simulink model "PHIL_DHS_DQ_Control"  (R2019b)
settings: Solver=VariableStepAuto  StartTime=0.0  StopTime=00.5  RelTol=1e-3
undefined symbols (not defined in the file): Apd_i_dhs, Apd_u_dhs, C_dhs, f_sw_dhs, L_dhs, Tid_i_dhs, Tid_u_dhs, U_DC
libraries: coordinate_transformations x8, simulink x4
settings Model: Creator=kissd  LastModifiedBy=kissd

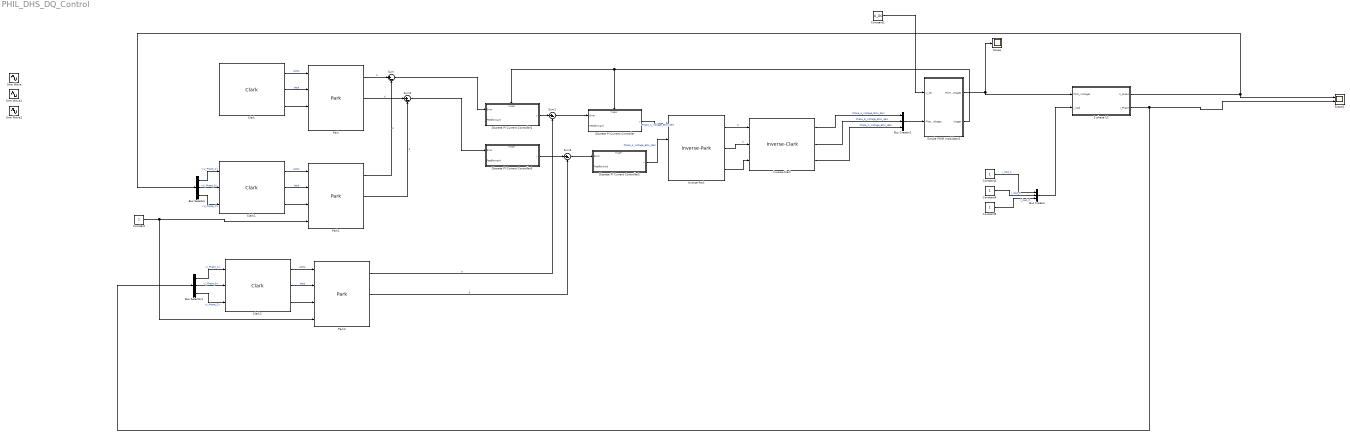
== system PHIL_DHS_DQ_Control ==
  3 phase LC : Subsystem
  Bus Creator : BusCreator  Inputs=3
  Bus Creator1 : BusCreator  Inputs=3
  Bus Selector : BusSelector  OutputSignals=U_Phase_A,U_Phase_B,U_Phase_C
  Bus Selector1 : BusSelector  OutputSignals=I_Phase_A,I_Phase_B,I_Phase_C
  Clark : coordinate_transformations/Clark  SystemSampleTime=-1  Latency=0  AutoFrameSizeCalculation=off
  Clark1 : coordinate_transformations/Clark  SystemSampleTime=-1  Latency=0  AutoFrameSizeCalculation=off
  Clark2 : coordinate_transformations/Clark  SystemSampleTime=-1  Latency=0  AutoFrameSizeCalculation=off
  Constant{,3..5} (4 alike) : Constant
  Constant1 : Constant  Value=U_DC
  Discrete PI Current Controller : Subsystem  AncestorBlock=controllers/Discrete PI Controller  mask(Continous PI Controller){Apd=Apd_i_dhs, Tid=Tid_i_dhs, fs=f_sw_dhs, UpperSat=U_DC, LowerSat=0}
      mask prompts: Apd "Proprotional Gain"; Tid "Integration Time"; fs "fsw"; UpperSat "Max. Saturation"; LowerSat "Min. Saturation"
      mask help: Continous PI Controller description.
  Discrete PI Current Controller1 : Subsystem  AncestorBlock=controllers/Discrete PI Controller  mask(Continous PI Controller){Apd=Apd_u_dhs, Tid=Tid_u_dhs, fs=f_sw_dhs, UpperSat=200, LowerSat=-200}
      mask prompts: Apd "Proprotional Gain"; Tid "Integration Time"; fs "fsw"; UpperSat "Max. Saturation"; LowerSat "Min. Saturation"
      mask help: Continous PI Controller description.
  Discrete PI Current Controller2 : Subsystem  AncestorBlock=controllers/Discrete PI Controller  mask(Continous PI Controller){Apd=Apd_i_dhs, Tid=Tid_i_dhs, fs=f_sw_dhs, UpperSat=U_DC, LowerSat=0}
      mask prompts: Apd "Proprotional Gain"; Tid "Integration Time"; fs "fsw"; UpperSat "Max. Saturation"; LowerSat "Min. Saturation"
      mask help: Continous PI Controller description.
  Discrete PI Current Controller3 : Subsystem  AncestorBlock=controllers/Discrete PI Controller  mask(Continous PI Controller){Apd=Apd_u_dhs, Tid=Tid_u_dhs, fs=f_sw_dhs, UpperSat=200, LowerSat=-200}
      mask prompts: Apd "Proprotional Gain"; Tid "Integration Time"; fs "fsw"; UpperSat "Max. Saturation"; LowerSat "Min. Saturation"
      mask help: Continous PI Controller description.
  Inverse-Clark : coordinate_transformations/Inverse-Clark  SystemSampleTime=-1  Latency=0  AutoFrameSizeCalculation=off
  Inverse-Park : coordinate_transformations/Inverse-Park  SystemSampleTime=-1  Latency=0  AutoFrameSizeCalculation=off
  Park : coordinate_transformations/Park  SystemSampleTime=-1  Latency=0  AutoFrameSizeCalculation=off
  Park1 : coordinate_transformations/Park  SystemSampleTime=-1  Latency=0  AutoFrameSizeCalculation=off
  Park2 : coordinate_transformations/Park  SystemSampleTime=-1  Latency=0  AutoFrameSizeCalculation=off
  Scope : Scope
  Scope2 : Scope  NumInputPorts=2
  Simple PWM modulator2 : Subsystem  AncestorBlock=controllers/Simple PWM modulator
  Sine Wave : Sin  SampleTime=0
  Sine Wave1 : Sin  SampleTime=0
  Sine Wave2 : Sin  SampleTime=0
  Sum{,1..3} (4 alike) : Sum  Inputs=|+-
  wires:
  Constant1/1 -> Simple PWM modulator2/1(U_DC)
  Inverse-Clark/3 -> Bus Creator1/3  "Phase_C_Voltage_EMU_dem"
  Inverse-Clark/2 -> Bus Creator1/2  "Phase_B_Voltage_EMU_dem"
  Sum1/1 -> Discrete PI Current Controller/1(Error)
  Inverse-Clark/1 -> Bus Creator1/1  "Phase_A_Voltage_EMU_dem"
  Simple PWM modulator2/1(PWM_Voltages) -> Scope/1, 3 phase LC/1(PWM_Voltages)
  Bus Creator1/1 -> Simple PWM modulator2/2(Phase_Voltages)
  Simple PWM modulator2/2(trigger) -> Discrete PI Current Controller1/Trigger, Discrete PI Current Controller/Trigger
  Discrete PI Current Controller1/1(y) -> Sum1/1
  Sum/1 -> Discrete PI Current Controller1/1(Error)
  Clark/1 -> Park/1  "alpha"
  Clark/2 -> Park/2  "beta"
  Clark/3 -> Park/3
  3 phase LC/2(I_Phase) -> Bus Selector1/1, Scope2/2
  3 phase LC/1(U_phase) -> Scope2/1, Bus Selector/1
  Constant3/1 -> Bus Creator/1  "I_load_A"
  Constant4/1 -> Bus Creator/2  "I_load_B"
  Constant5/1 -> Bus Creator/3  "I_load_C"
  Bus Creator/1 -> 3 phase LC/2(I_load)
  Inverse-Park/1 -> Inverse-Clark/1  "d"
  Inverse-Park/2 -> Inverse-Clark/2  "q"
  Inverse-Park/3 -> Inverse-Clark/3
  Park/1 -> Sum/1  "d"
  Discrete PI Current Controller/1(y) -> Inverse-Park/1  "Phase_A_Voltage_EMU_dem"
  Sum2/1 -> Discrete PI Current Controller3/1(Error)
  Discrete PI Current Controller3/1(y) -> Sum3/1
  Park/2 -> Sum2/1  "d"
  Sum3/1 -> Discrete PI Current Controller2/1(Error)
  Discrete PI Current Controller2/1(y) -> Inverse-Park/2  "Phase_A_Voltage_EMU_dem"
  Clark1/3 -> Park1/3
  Clark1/1 -> Park1/1  "alpha"
  Clark1/2 -> Park1/2  "beta"
  Clark2/3 -> Park2/3
  Clark2/1 -> Park2/1  "alpha"
  Clark2/2 -> Park2/2  "beta"
  Bus Selector/1 -> Clark1/1  "<U_Phase_A>"
  Bus Selector/2 -> Clark1/2  "<U_Phase_B>"
  Bus Selector/3 -> Clark1/3  "<U_Phase_C>"
  Bus Selector1/1 -> Clark2/1  "<I_Phase_A>"
  Bus Selector1/2 -> Clark2/2  "<I_Phase_B>"
  Bus Selector1/3 -> Clark2/3  "<I_Phase_C>"
  Constant/1 -> Park2/4, Park1/4
  Park1/1 -> Sum/2  "d"
  Park1/2 -> Sum2/2  "d"
  Park2/1 -> Sum1/2  "d"
  Park2/2 -> Sum3/2  "d"

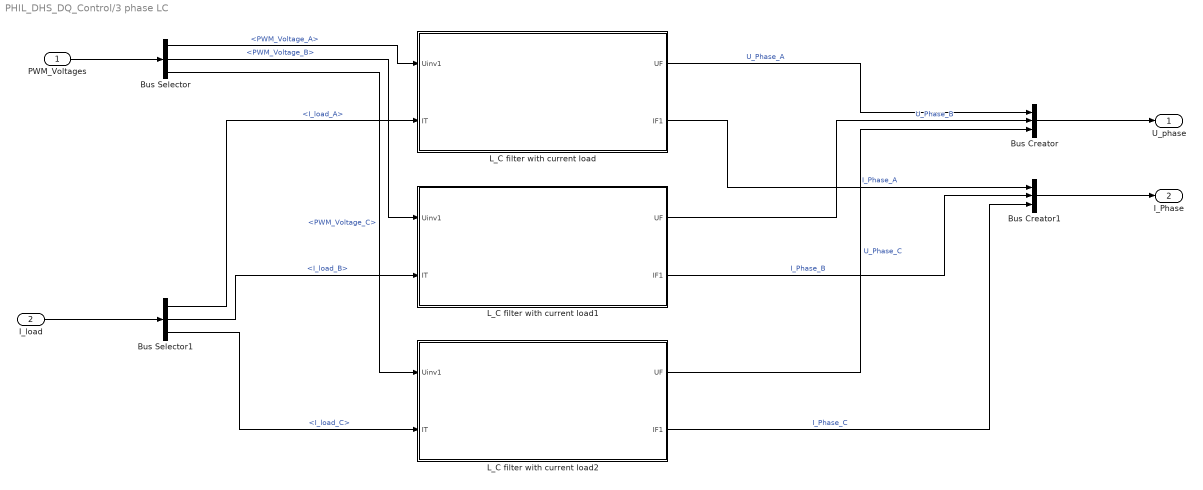
== system PHIL_DHS_DQ_Control/3 phase LC ==
  PWM_Voltages : Inport
  I_load : Inport  Port=2
  Bus Creator : BusCreator  Inputs=3
  Bus Creator1 : BusCreator  Inputs=3
  Bus Selector : BusSelector  OutputSignals=PWM_Voltage_A,PWM_Voltage_B,PWM_Voltage_C
  Bus Selector1 : BusSelector  OutputSignals=I_load_A,I_load_B,I_load_C
  L_C filter with current load : Subsystem
  L_C filter with current load1 : Subsystem
  L_C filter with current load2 : Subsystem
  U_phase : Outport
  I_Phase : Outport  Port=2
  wires:
  L_C filter with current load1/1(UF) -> Bus Creator/2  "U_Phase_B"
  L_C filter with current load2/1(UF) -> Bus Creator/3  "U_Phase_C"
  Bus Selector1/3 -> L_C filter with current load2/2(IT)  "<I_load_C>"
  L_C filter with current load1/2(IF1) -> Bus Creator1/2  "I_Phase_B"
  L_C filter with current load2/2(IF1) -> Bus Creator1/3  "I_Phase_C"
  PWM_Voltages/1 -> Bus Selector/1
  Bus Selector/1 -> L_C filter with current load/1(Uinv1)  "<PWM_Voltage_A>"
  Bus Selector/2 -> L_C filter with current load1/1(Uinv1)  "<PWM_Voltage_B>"
  Bus Selector/3 -> L_C filter with current load2/1(Uinv1)  "<PWM_Voltage_C>"
  Bus Creator/1 -> U_phase/1
  L_C filter with current load/1(UF) -> Bus Creator/1  "U_Phase_A"
  L_C filter with current load/2(IF1) -> Bus Creator1/1  "I_Phase_A"
  Bus Creator1/1 -> I_Phase/1
  I_load/1 -> Bus Selector1/1
  Bus Selector1/1 -> L_C filter with current load/2(IT)  "<I_load_A>"
  Bus Selector1/2 -> L_C filter with current load1/2(IT)  "<I_load_B>"

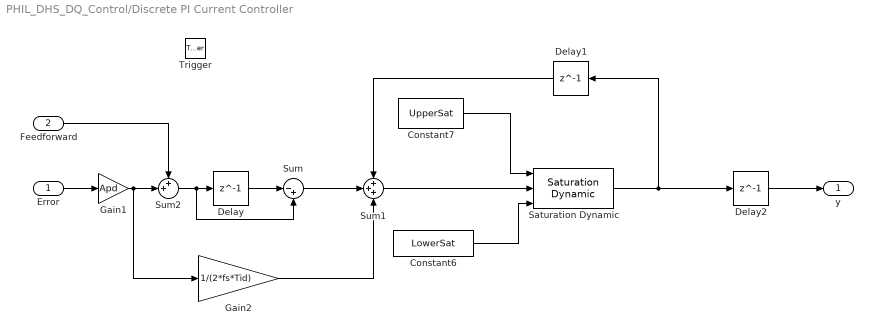
== system PHIL_DHS_DQ_Control/Discrete PI Current Controller ==
  Error : Inport
  Feedforward : Inport  Port=2
  Trigger : TriggerPort  TriggerType=either  VariantControl=Variant  PortDimensions=1
  Constant6 : Constant  Value=LowerSat
  Constant7 : Constant  Value=UpperSat
  Delay : Delay  DelayLength=1
  Delay1 : Delay  DelayLength=1
  Delay2 : Delay  DelayLength=1
  Gain1 : Gain  Gain=Apd
  Gain2 : Gain  Gain=1/(2*fs*Tid)
  Saturation Dynamic : simulink/Discontinuities/Saturation Dynamic  OutMin=[]  OutMax=[]  OutDataTypeStr=Inherit: Same as second input  OutDataType=fixdt(1, 16)  OutScaling=2^-10  DoSatur=off
  Sum : Sum  Inputs=|-+
  Sum1 : Sum  Inputs=+++
  Sum2 : Sum  Inputs=++|
  y : Outport
  wires:
  Error/1 -> Gain1/1
  Gain1/1 -> Sum2/2, Gain2/1
  Sum1/1 -> Saturation Dynamic/2
  Saturation Dynamic/1 -> Delay1/1, Delay2/1
  Constant7/1 -> Saturation Dynamic/1
  Constant6/1 -> Saturation Dynamic/3
  Delay/1 -> Sum/1
  Sum/1 -> Sum1/2
  Gain2/1 -> Sum1/3
  Delay1/1 -> Sum1/1
  Delay2/1 -> y/1
  Sum2/1 -> Sum/2, Delay/1
  Feedforward/1 -> Sum2/1

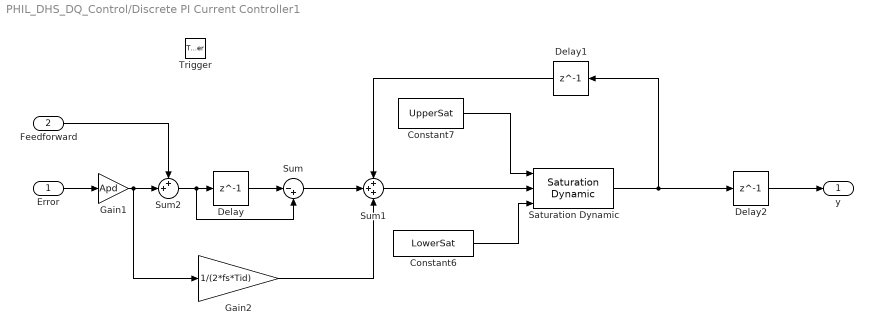
== system PHIL_DHS_DQ_Control/Discrete PI Current Controller1 ==
  Error : Inport
  Feedforward : Inport  Port=2
  Trigger : TriggerPort  TriggerType=either  VariantControl=Variant  PortDimensions=1
  Constant6 : Constant  Value=LowerSat
  Constant7 : Constant  Value=UpperSat
  Delay : Delay  DelayLength=1
  Delay1 : Delay  DelayLength=1
  Delay2 : Delay  DelayLength=1
  Gain1 : Gain  Gain=Apd
  Gain2 : Gain  Gain=1/(2*fs*Tid)
  Saturation Dynamic : simulink/Discontinuities/Saturation Dynamic  OutMin=[]  OutMax=[]  OutDataTypeStr=Inherit: Same as second input  OutDataType=fixdt(1, 16)  OutScaling=2^-10  DoSatur=off
  Sum : Sum  Inputs=|-+
  Sum1 : Sum  Inputs=+++
  Sum2 : Sum  Inputs=++|
  y : Outport
  wires:
  Error/1 -> Gain1/1
  Gain1/1 -> Sum2/2, Gain2/1
  Sum1/1 -> Saturation Dynamic/2
  Saturation Dynamic/1 -> Delay1/1, Delay2/1
  Constant7/1 -> Saturation Dynamic/1
  Constant6/1 -> Saturation Dynamic/3
  Delay/1 -> Sum/1
  Sum/1 -> Sum1/2
  Gain2/1 -> Sum1/3
  Delay1/1 -> Sum1/1
  Delay2/1 -> y/1
  Sum2/1 -> Sum/2, Delay/1
  Feedforward/1 -> Sum2/1

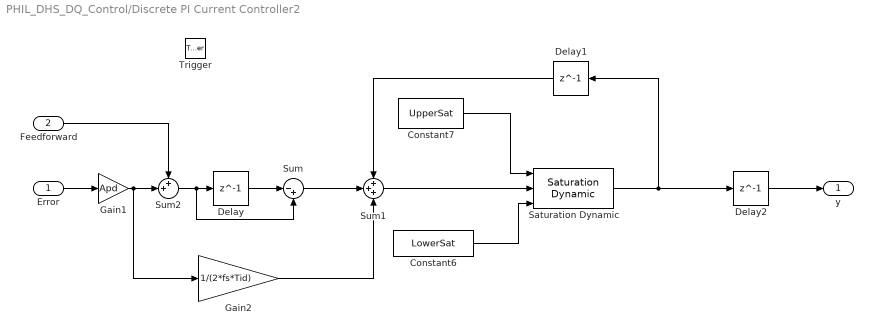
== system PHIL_DHS_DQ_Control/Discrete PI Current Controller2 ==
  Error : Inport
  Feedforward : Inport  Port=2
  Trigger : TriggerPort  TriggerType=either  VariantControl=Variant  PortDimensions=1
  Constant6 : Constant  Value=LowerSat
  Constant7 : Constant  Value=UpperSat
  Delay : Delay  DelayLength=1
  Delay1 : Delay  DelayLength=1
  Delay2 : Delay  DelayLength=1
  Gain1 : Gain  Gain=Apd
  Gain2 : Gain  Gain=1/(2*fs*Tid)
  Saturation Dynamic : simulink/Discontinuities/Saturation Dynamic  OutMin=[]  OutMax=[]  OutDataTypeStr=Inherit: Same as second input  OutDataType=fixdt(1, 16)  OutScaling=2^-10  DoSatur=off
  Sum : Sum  Inputs=|-+
  Sum1 : Sum  Inputs=+++
  Sum2 : Sum  Inputs=++|
  y : Outport
  wires:
  Error/1 -> Gain1/1
  Gain1/1 -> Sum2/2, Gain2/1
  Sum1/1 -> Saturation Dynamic/2
  Saturation Dynamic/1 -> Delay1/1, Delay2/1
  Constant7/1 -> Saturation Dynamic/1
  Constant6/1 -> Saturation Dynamic/3
  Delay/1 -> Sum/1
  Sum/1 -> Sum1/2
  Gain2/1 -> Sum1/3
  Delay1/1 -> Sum1/1
  Delay2/1 -> y/1
  Sum2/1 -> Sum/2, Delay/1
  Feedforward/1 -> Sum2/1

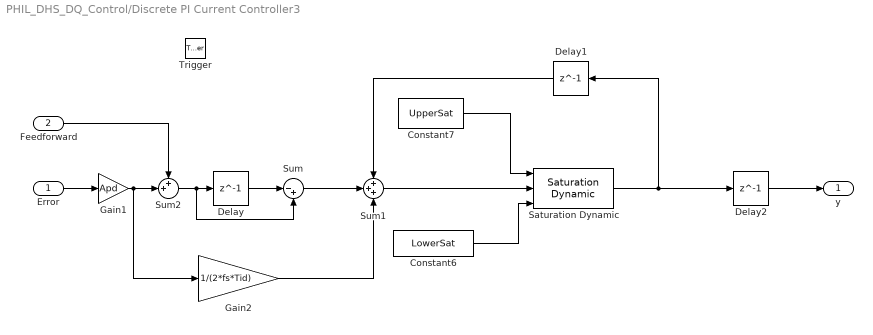
== system PHIL_DHS_DQ_Control/Discrete PI Current Controller3 ==
  Error : Inport
  Feedforward : Inport  Port=2
  Trigger : TriggerPort  TriggerType=either  VariantControl=Variant  PortDimensions=1
  Constant6 : Constant  Value=LowerSat
  Constant7 : Constant  Value=UpperSat
  Delay : Delay  DelayLength=1
  Delay1 : Delay  DelayLength=1
  Delay2 : Delay  DelayLength=1
  Gain1 : Gain  Gain=Apd
  Gain2 : Gain  Gain=1/(2*fs*Tid)
  Saturation Dynamic : simulink/Discontinuities/Saturation Dynamic  OutMin=[]  OutMax=[]  OutDataTypeStr=Inherit: Same as second input  OutDataType=fixdt(1, 16)  OutScaling=2^-10  DoSatur=off
  Sum : Sum  Inputs=|-+
  Sum1 : Sum  Inputs=+++
  Sum2 : Sum  Inputs=++|
  y : Outport
  wires:
  Error/1 -> Gain1/1
  Gain1/1 -> Sum2/2, Gain2/1
  Sum1/1 -> Saturation Dynamic/2
  Saturation Dynamic/1 -> Delay1/1, Delay2/1
  Constant7/1 -> Saturation Dynamic/1
  Constant6/1 -> Saturation Dynamic/3
  Delay/1 -> Sum/1
  Sum/1 -> Sum1/2
  Gain2/1 -> Sum1/3
  Delay1/1 -> Sum1/1
  Delay2/1 -> y/1
  Sum2/1 -> Sum/2, Delay/1
  Feedforward/1 -> Sum2/1

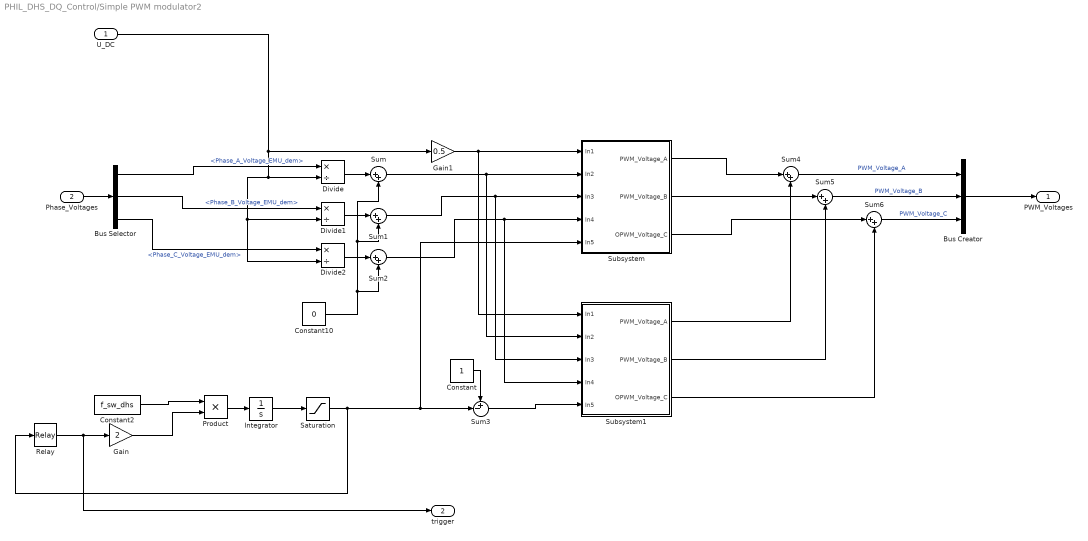
== system PHIL_DHS_DQ_Control/Simple PWM modulator2 ==
  U_DC : Inport
  Phase_Voltages : Inport  Port=2
  Bus Creator : BusCreator  Inputs=3
  Bus Selector : BusSelector  OutputSignals=Phase_A_Voltage_EMU_dem,Phase_B_Voltage_EMU_dem,Phase_C_Voltage_EMU_dem
  Constant : Constant
  Constant10 : Constant  Value=0
  Constant2 : Constant  Value=f_sw_dhs
  Divide : Product  Inputs=*/
  Divide1 : Product  Inputs=*/
  Divide2 : Product  Inputs=*/
  Gain : Gain  Gain=2
  Gain1 : Gain  Gain=0.5
  Integrator : Integrator
  Product : Product
  Relay : Relay  OnSwitchValue=1  OffSwitchValue=0  OnOutputValue=-1  OffOutputValue=1
  Saturation : Saturate  UpperLimit=1  LowerLimit=0
  Subsystem : Subsystem
  Subsystem1 : Subsystem
  Sum{,1..2,4..6} (6 alike) : Sum  Inputs=|++
  Sum3 : Sum  Inputs=+-|
  PWM_Voltages : Outport
  trigger : Outport  Port=2
  wires:
  Constant2/1 -> Product/1
  Product/1 -> Integrator/1
  Integrator/1 -> Saturation/1
  Divide1/1 -> Sum1/1
  Saturation/1 -> Subsystem/5(In5), Sum3/2, Relay/1
  Relay/1 -> trigger/1, Gain/1
  Constant10/1 -> Sum2/2, Sum1/2, Sum/2
  Bus Selector/1 -> Divide/1  "<Phase_A_Voltage_EMU_dem>"
  Gain/1 -> Product/2
  Divide2/1 -> Sum2/1
  Divide/1 -> Sum/1
  Bus Selector/3 -> Divide2/1  "<Phase_C_Voltage_EMU_dem>"
  Bus Selector/2 -> Divide1/1  "<Phase_B_Voltage_EMU_dem>"
  Phase_Voltages/1 -> Bus Selector/1
  Bus Creator/1 -> PWM_Voltages/1
  Constant/1 -> Sum3/1
  Sum/1 -> Subsystem1/2(In2), Subsystem/2(In2)
  Sum1/1 -> Subsystem1/3(In3), Subsystem/3(In3)
  Sum2/1 -> Subsystem1/4(In4), Subsystem/4(In4)
  Sum3/1 -> Subsystem1/5(In5)
  Sum4/1 -> Bus Creator/1  "PWM_Voltage_A"
  Subsystem/1(PWM_Voltage_A) -> Sum4/1
  Subsystem1/1(PWM_Voltage_A) -> Sum4/2
  Sum5/1 -> Bus Creator/2  "PWM_Voltage_B"
  Subsystem/2(PWM_Voltage_B) -> Sum5/1
  Subsystem1/2(PWM_Voltage_B) -> Sum5/2
  Sum6/1 -> Bus Creator/3  "PWM_Voltage_C"
  Subsystem/3(OPWM_Voltage_C) -> Sum6/1
  Subsystem1/3(OPWM_Voltage_C) -> Sum6/2
  U_DC/1 -> Gain1/1, Divide2/2, Divide1/2, Divide/2
  Gain1/1 -> Subsystem1/1(In1), Subsystem/1(In1)

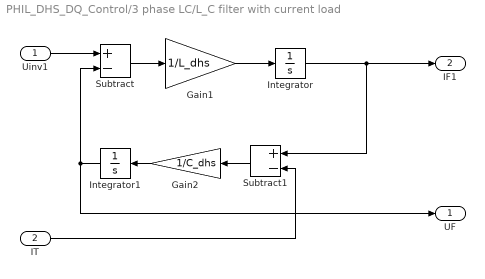
== system PHIL_DHS_DQ_Control/3 phase LC/L_C filter with current load ==
  Uinv1 : Inport
  IT : Inport  Port=2
  Gain1 : Gain  Gain=1/L_dhs
  Gain2 : Gain  Gain=1/C_dhs
  Integrator : Integrator
  Integrator1 : Integrator
  Subtract : Sum  Inputs=+-
  Subtract1 : Sum  Inputs=+-
  UF : Outport
  IF1 : Outport  Port=2
  wires:
  Integrator1/1 -> UF/1, Subtract/2
  Subtract/1 -> Gain1/1
  Gain1/1 -> Integrator/1
  Integrator/1 -> Subtract1/1, IF1/1
  IT/1 -> Subtract1/2
  Gain2/1 -> Integrator1/1
  Uinv1/1 -> Subtract/1
  Subtract1/1 -> Gain2/1

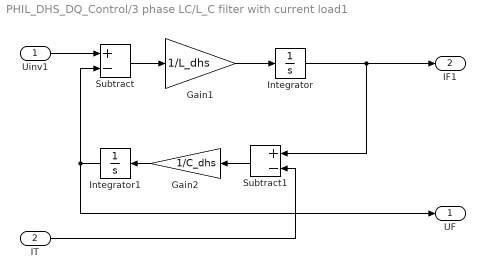
== system PHIL_DHS_DQ_Control/3 phase LC/L_C filter with current load1 ==
  Uinv1 : Inport
  IT : Inport  Port=2
  Gain1 : Gain  Gain=1/L_dhs
  Gain2 : Gain  Gain=1/C_dhs
  Integrator : Integrator
  Integrator1 : Integrator
  Subtract : Sum  Inputs=+-
  Subtract1 : Sum  Inputs=+-
  UF : Outport
  IF1 : Outport  Port=2
  wires:
  Integrator1/1 -> UF/1, Subtract/2
  Subtract/1 -> Gain1/1
  Gain1/1 -> Integrator/1
  Integrator/1 -> Subtract1/1, IF1/1
  IT/1 -> Subtract1/2
  Gain2/1 -> Integrator1/1
  Uinv1/1 -> Subtract/1
  Subtract1/1 -> Gain2/1

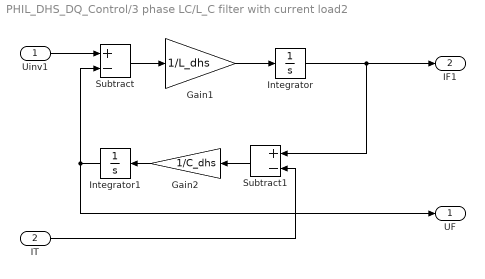
== system PHIL_DHS_DQ_Control/3 phase LC/L_C filter with current load2 ==
  Uinv1 : Inport
  IT : Inport  Port=2
  Gain1 : Gain  Gain=1/L_dhs
  Gain2 : Gain  Gain=1/C_dhs
  Integrator : Integrator
  Integrator1 : Integrator
  Subtract : Sum  Inputs=+-
  Subtract1 : Sum  Inputs=+-
  UF : Outport
  IF1 : Outport  Port=2
  wires:
  Integrator1/1 -> UF/1, Subtract/2
  Subtract/1 -> Gain1/1
  Gain1/1 -> Integrator/1
  Integrator/1 -> Subtract1/1, IF1/1
  IT/1 -> Subtract1/2
  Gain2/1 -> Integrator1/1
  Uinv1/1 -> Subtract/1
  Subtract1/1 -> Gain2/1

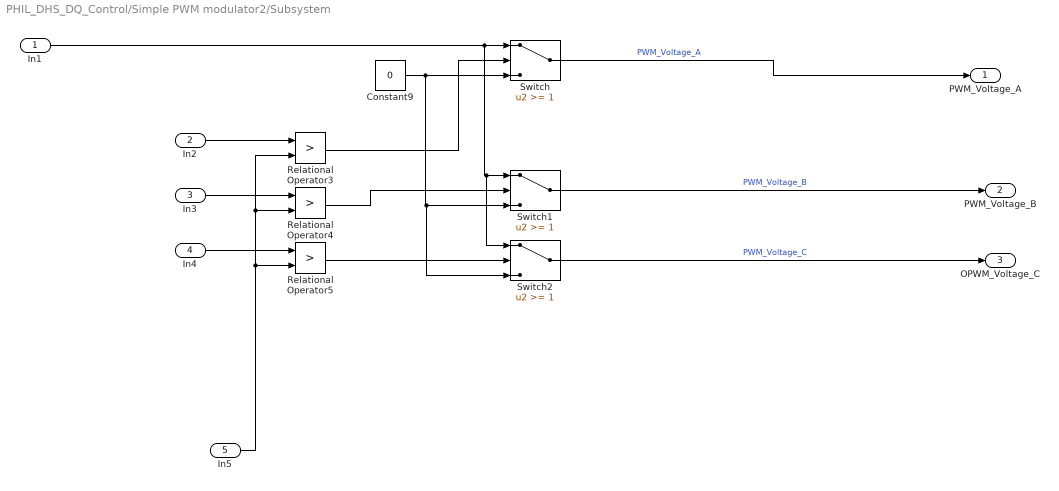
== system PHIL_DHS_DQ_Control/Simple PWM modulator2/Subsystem ==
  In1 : Inport
  In2 : Inport  Port=2
  In3 : Inport  Port=3
  In4 : Inport  Port=4
  In5 : Inport  Port=5
  Constant9 : Constant  Value=0
  Relational Operator3 : RelationalOperator  Operator=>  OutDataTypeStr=boolean  RndMeth=Simplest
  Relational Operator4 : RelationalOperator  Operator=>  OutDataTypeStr=boolean  RndMeth=Simplest
  Relational Operator5 : RelationalOperator  Operator=>  OutDataTypeStr=boolean  RndMeth=Simplest
  Switch : Switch  Threshold=1
  Switch1 : Switch  Threshold=1
  Switch2 : Switch  Threshold=1
  PWM_Voltage_A : Outport
  PWM_Voltage_B : Outport  Port=2
  OPWM_Voltage_C : Outport  Port=3
  wires:
  Relational Operator4/1 -> Switch1/2
  In5/1 -> Relational Operator3/2, Relational Operator4/2, Relational Operator5/2
  Constant9/1 -> Switch2/3, Switch1/3, Switch/3
  Relational Operator3/1 -> Switch/2
  In3/1 -> Relational Operator4/1
  Relational Operator5/1 -> Switch2/2
  Switch/1 -> PWM_Voltage_A/1  "PWM_Voltage_A"
  In1/1 -> Switch2/1, Switch1/1, Switch/1
  In2/1 -> Relational Operator3/1
  In4/1 -> Relational Operator5/1
  Switch1/1 -> PWM_Voltage_B/1  "PWM_Voltage_B"
  Switch2/1 -> OPWM_Voltage_C/1  "PWM_Voltage_C"

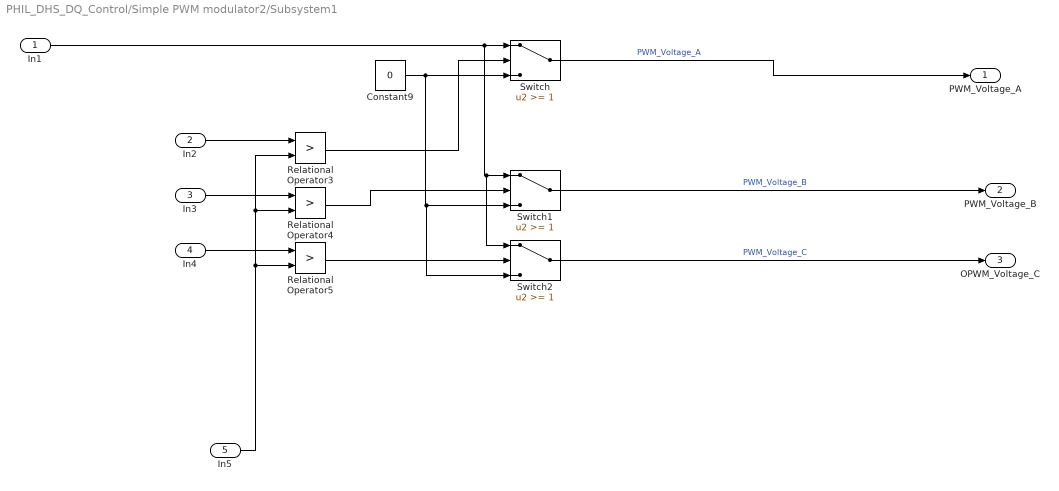
== system PHIL_DHS_DQ_Control/Simple PWM modulator2/Subsystem1 ==
  In1 : Inport
  In2 : Inport  Port=2
  In3 : Inport  Port=3
  In4 : Inport  Port=4
  In5 : Inport  Port=5
  Constant9 : Constant  Value=0
  Relational Operator3 : RelationalOperator  Operator=>  OutDataTypeStr=boolean  RndMeth=Simplest
  Relational Operator4 : RelationalOperator  Operator=>  OutDataTypeStr=boolean  RndMeth=Simplest
  Relational Operator5 : RelationalOperator  Operator=>  OutDataTypeStr=boolean  RndMeth=Simplest
  Switch : Switch  Threshold=1
  Switch1 : Switch  Threshold=1
  Switch2 : Switch  Threshold=1
  PWM_Voltage_A : Outport
  PWM_Voltage_B : Outport  Port=2
  OPWM_Voltage_C : Outport  Port=3
  wires:
  Relational Operator4/1 -> Switch1/2
  In5/1 -> Relational Operator3/2, Relational Operator4/2, Relational Operator5/2
  Constant9/1 -> Switch2/3, Switch1/3, Switch/3
  Relational Operator3/1 -> Switch/2
  In3/1 -> Relational Operator4/1
  Relational Operator5/1 -> Switch2/2
  Switch/1 -> PWM_Voltage_A/1  "PWM_Voltage_A"
  In1/1 -> Switch2/1, Switch1/1, Switch/1
  In2/1 -> Relational Operator3/1
  In4/1 -> Relational Operator5/1
  Switch1/1 -> PWM_Voltage_B/1  "PWM_Voltage_B"
  Switch2/1 -> OPWM_Voltage_C/1  "PWM_Voltage_C"
